simulink model "FeedbackLinearization"  (R2018a)
settings: Solver=ode45  StartTime=0.0  StopTime=20  MaxStep=1e-4  RelTol=1e-4  EnableMultiTasking=on
values from neighbouring files (symbols this model uses):
  a = 0.025    [variables.m]
  alpha = (3*Pa)/(4*a*Pb)    (= 3.41538461538)    [variables.m]
  g = 9.81    [variables.m]
  Pa = 1.184    [variables.m]
  Pb = 10.4    [variables.m]
settings Model: Creator=Gabriel  LastModifiedBy=Aluno
settings SolverCC: ZeroCrossControl=DisableAll
settings DataIOCC: LimitDataPoints=on  SaveFormat=Array
settings OptimizationCC: LifeSpan=inf
settings DebuggingCC: UnderspecifiedInitializationDetection=Classic  MergeDetectMultiDrivingBlocksExec=none  SolverPrmCheckMsg=warning  StateNameClashWarn=warning  SFUnexpectedBacktrackingDiag=warning  SFNoUnconditionalDefaultTransitionDiag=warning  SFExecutionAtInitializationDiag=none
settings HardwareCC: ProdBitPerPointer=32  ProdBitPerSizeT=32  ProdBitPerPtrDiffT=32  ProdLargestAtomicFloat=None  ProdIntDivRoundTo=Undefined  ProdEndianess=Unspecified  ProdWordSize=32  ProdHWDeviceType=32-bit Generic
settings ModelReferenceCC: PropagateSignalLabelsOutOfModel=off
settings CodeAppCC: StateflowObjectComments=on
settings GRTTargetCC: TargetLangStandard=C89/C90 (ANSI)  GeneratePreprocessorConditionals=Disable all
settings ConfigComp: CovMetricSettings=dw  CovHtmlReporting=on  CovSaveCumulativeToWorkspaceVar=on  CovSaveSingleToWorkspaceVar=on  CovExternalEMLEnable=off

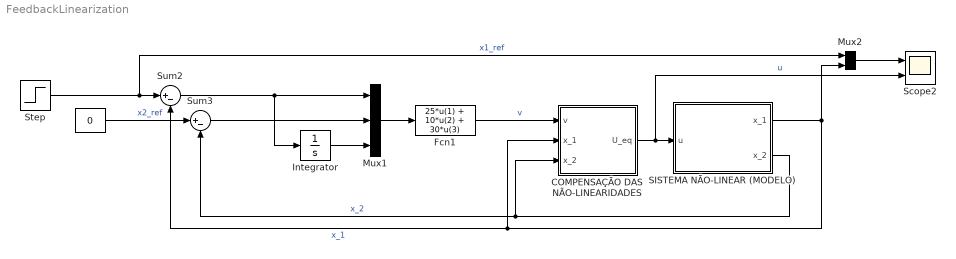
== system FeedbackLinearization ==
  "   " : Constant  Value=0
  COMPENSAÇÃO DAS NÃO-LINEARIDADES : Subsystem
  Fcn1 : Fcn  Expr=25*u(1) + 10*u(2) + 30*u(3)
  Integrator : Integrator
  Mux1 : Mux  Inputs=3
  Mux2 : Mux  Inputs=2
  SISTEMA NÃO-LINEAR (MODELO) : Subsystem
  Scope2 : Scope  NumInputPorts=2
  Step : Step  Time=0  Before=0.15  After=0.6  SampleTime=0
  Sum2 : Sum  Inputs=|+-
  Sum3 : Sum  Inputs=|+-
  wires:
  SISTEMA NÃO-LINEAR (MODELO)/1(x_1) -> Mux2/2, Sum2/2, COMPENSAÇÃO DAS NÃO-LINEARIDADES/2(x_1)  "x_1"
  Fcn1/1 -> COMPENSAÇÃO DAS NÃO-LINEARIDADES/1(v)  "v"
  SISTEMA NÃO-LINEAR (MODELO)/2(x_2) -> Sum3/2, COMPENSAÇÃO DAS NÃO-LINEARIDADES/3(x_2)  "x_2"
  "   "/1 -> Sum3/1  "x2_ref"
  COMPENSAÇÃO DAS NÃO-LINEARIDADES/1(U_eq) -> SISTEMA NÃO-LINEAR (MODELO)/1(u), Scope2/2  "u"
  Step/1 -> Mux2/1, Sum2/1  "x1_ref"
  Sum3/1 -> Mux1/2
  Sum2/1 -> Integrator/1, Mux1/1
  Mux1/1 -> Fcn1/1
  Mux2/1 -> Scope2/1
  Integrator/1 -> Mux1/3

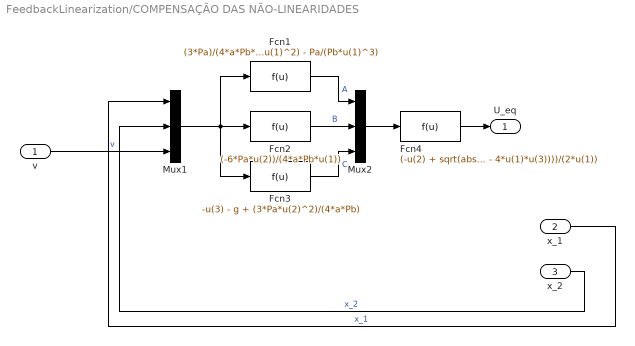
== system FeedbackLinearization/COMPENSAÇÃO DAS NÃO-LINEARIDADES ==
  v : Inport
  x_1 : Inport  Port=2
  x_2 : Inport  Port=3
  Fcn1 : Fcn  Expr=(3*Pa)/(4*a*Pb*u(1)^2) - Pa/(Pb*u(1)^3)
  Fcn2 : Fcn  Expr=(-6*Pa*u(2))/(4*a*Pb*u(1))
  Fcn3 : Fcn  Expr=-u(3) - g + (3*Pa*u(2)^2)/(4*a*Pb)
  Fcn4 : Fcn  Expr=(-u(2) + sqrt(abs(u(2)^2 - 4*u(1)*u(3))))/(2*u(1))
  Mux1 : Mux  Inputs=3
  Mux2 : Mux  Inputs=3
  U_eq : Outport
  wires:
  x_2/1 -> Mux1/2  "x_2"
  x_1/1 -> Mux1/1  "x_1"
  v/1 -> Mux1/3  "v"
  Fcn1/1 -> Mux2/1  "A"
  Fcn2/1 -> Mux2/2  "B"
  Fcn3/1 -> Mux2/3  "C"
  Mux2/1 -> Fcn4/1
  Fcn4/1 -> U_eq/1
  Mux1/1 -> Fcn1/1, Fcn2/1, Fcn3/1

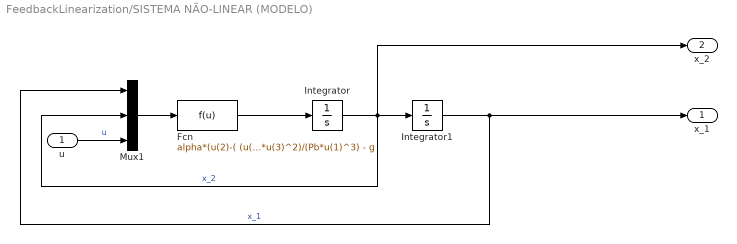
== system FeedbackLinearization/SISTEMA NÃO-LINEAR (MODELO) ==
  u : Inport
  Fcn : Fcn  Expr=alpha*(u(2)-( (u(3))/u(1)) )^2 - (Pa*u(3)^2)/(Pb*u(1)^3) - g
  Integrator : Integrator
  Integrator1 : Integrator  InitialCondition=0.1  LimitOutput=on  UpperSaturationLimit=2  LowerSaturationLimit=0.001
  Mux1 : Mux  Inputs=3
  x_1 : Outport
  x_2 : Outport  Port=2
  wires:
  Fcn/1 -> Integrator/1
  Integrator/1 -> Mux1/2, x_2/1, Integrator1/1  "x_2"
  u/1 -> Mux1/3  "u"
  Mux1/1 -> Fcn/1
  Integrator1/1 -> Mux1/1, x_1/1  "x_1"
